simulink model "controlstructureforassignment"  (R2022b)
settings: Solver=ode45  StartTime=0.0  StopTime=300  RelTol=1e-6  EnableMultiTasking=on
values from neighbouring files (symbols this model uses):
  At = 63.6    [LAB.m]
  h10 = 14    [LAB.m]
  h20 = 14    [LAB.m]
  K_q = 10    [LAB.m]
  Ki = Tau/(Kp*lambda)    [LAB.m]
  Kp = 0.1572*Tau    (= 7.09706546275)    [LAB.m]
  Kr = 1    [LAB.m]
  Lc = 1    [LAB.m]
  point = [14, 14]    [LAB.m]
  u10 = u_1_init    [LAB.m]
  u20 = u_2_init    [LAB.m]
settings Model: Creator=magni246  LastModifiedBy=danisode
settings SolverCC: ZeroCrossAlgorithm=Non-adaptive  AlgebraicLoopSolver=TrustRegion
settings DataIOCC: LimitDataPoints=on  SaveFormat=Array  SignalLoggingSaveFormat=ModelDataLogs  ReturnWorkspaceOutputs=off
settings OptimizationCC: ExpressionDepthLimit=2147483647  InitFltsAndDblsToZero=on  LifeSpan=inf
settings DebuggingCC: UnderspecifiedInitializationDetection=Classic  MergeDetectMultiDrivingBlocksExec=none  SolverPrmCheckMsg=warning  FcnCallInpInsideContextMsg=warning  UnconnectedInputMsg=warning  UnconnectedOutputMsg=warning  UnconnectedLineMsg=warning  StateNameClashWarn=warning  SFUnexpectedBacktrackingDiag=warning  SFNoUnconditionalDefaultTransitionDiag=warning  SFExecutionAtInitializationDiag=none  SFMachineParentedDataDiag=warning  ArithmeticOperatorsInVariantConditions=warning
settings HardwareCC: ProdBitPerPointer=32  ProdBitPerSizeT=32  ProdBitPerPtrDiffT=32  ProdLargestAtomicFloat=None  ProdIntDivRoundTo=Undefined  ProdEndianess=Unspecified  ProdWordSize=32  ProdHWDeviceType=32-bit Generic
settings ModelReferenceCC: PropagateSignalLabelsOutOfModel=off
settings CodeAppCC: StateflowObjectComments=on
settings GRTTargetCC: TargetLangStandard=C89/C90 (ANSI)  CombineOutputUpdateFcns=off  GRTInterface=on
settings ConfigComp: CovMetricSettings=dw  CovSaveCumulativeToWorkspaceVar=on  CovSaveSingleToWorkspaceVar=on

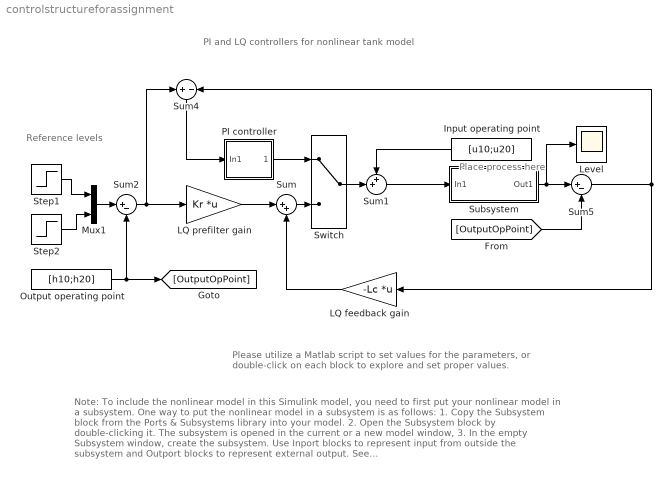
== system controlstructureforassignment ==
  note: Reference
      | levels
  note: Note: To include the nonlinear model in this Simulink model,
      | you need to first put your nonlinear model in a subsystem.
      |
      | One way to put the nonlinear model in a subsystem is as follows:
      |    1.  Copy the Subsystem block from the Ports & Subsystems library into your model.
      |    2. Open the Subsystem block by double-clicking it.
      |       The subsystem is opened in the current or a new model window,
      |    3. In the empty Subsystem window, create the subsystem.
      | Use Inport blocks to represent input from outside the subsystem
      | and Outport blocks to represent external output.
      |
      | See http://www.mathworks.com/access/helpdesk/help/toolbox/simulink/index.html?/access/helpdesk/help/toolbox/simulink/ug/f4-53172.html
  note: Please utilize a Matlab script to set values for the parameters,
      | or double-click on each block to explore and set proper values.
  note: PI and LQ controllers for nonlinear tank model
  note: Place process
      | here
  Input operating point : Constant  Value=[u10;u20]
  LQ feedback gain : Gain  Gain=-Lc  Multiplication=Matrix(K*u)
  LQ prefilter gain : Gain  Gain=Kr  Multiplication=Matrix(K*u)
  Level : Scope
  Mux1 : Mux  Inputs=2
  "Output operating point " : Constant  Value=[h10;h20]
  PI controller : Subsystem
  Step1 : Step  Time=100  Before=h10  After=h10+2  SampleTime=0
  Step2 : Step  Time=100  Before=h20  After=h20  SampleTime=0
  Subsystem : Subsystem
  Sum : Sum  Inputs=|++
  Sum1 : Sum  Inputs=++|
  Sum2 : Sum  Inputs=|+-
  Sum4 : Sum  Inputs=+-
  Sum5 : Sum  Inputs=|+-
  "Switch " : ManualSwitch
  wires:
  LQ prefilter gain/1 -> Sum/1
  LQ feedback gain/1 -> Sum/2
  Sum/1 -> "Switch "/2
  Step2/1 -> Mux1/2
  Step1/1 -> Mux1/1
  Sum1/1 -> Subsystem/1(In1)
  Sum2/1 -> LQ prefilter gain/1, Sum4/1
  Mux1/1 -> Sum2/1
  "Output operating point "/1 -> Sum2/2, [OutputOpPoint]
  PI controller/1(Out1) -> "Switch "/1
  Sum4/1 -> PI controller/1(In1)
  [OutputOpPoint] -> Sum5/2
  Subsystem/1(Out1) -> Sum5/1, Level/1
  Sum5/1 -> LQ feedback gain/1, Sum4/2
  "Switch "/1 -> Sum1/2
  Input operating point/1 -> Sum1/1

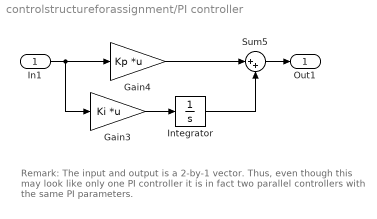
== system controlstructureforassignment/PI controller ==
  note: Remark:  The input and output is a 2-by-1 vector.  Thus, even though
      | this may look like only one PI controller it is in fact two parallel
      | controllers with the same PI parameters.
  In1 : Inport
  Gain3 : Gain  Gain=Ki  Multiplication=Matrix(K*u)
  Gain4 : Gain  Gain=Kp  Multiplication=Matrix(K*u)
  Integrator : Integrator  LimitOutput=on  UpperSaturationLimit=10  LowerSaturationLimit=-10
  Sum5 : Sum  Inputs=|++
  Out1 : Outport
  wires:
  In1/1 -> Gain4/1, Gain3/1
  Gain4/1 -> Sum5/1
  Sum5/1 -> Out1/1
  Integrator/1 -> Sum5/2
  Gain3/1 -> Integrator/1

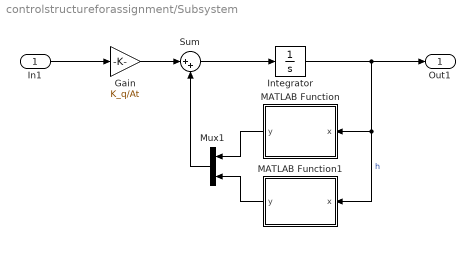
== system controlstructureforassignment/Subsystem ==
  In1 : Inport
  Gain : Gain  Gain=K_q/At
  Integrator : Integrator  InitialCondition=point
  MATLAB Function : MATLAB Function  TreatAsAtomicUnit=on
  MATLAB Function1 : MATLAB Function  TreatAsAtomicUnit=on
  Mux1 : Mux  Inputs=2
  Sum : Sum  Inputs=|++
  Out1 : Outport
  wires:
  Integrator/1 -> Out1/1, MATLAB Function1/1(x), MATLAB Function/1(x)  "h"
  In1/1 -> Gain/1
  Mux1/1 -> Sum/2
  MATLAB Function1/1(y) -> Mux1/2
  MATLAB Function/1(y) -> Mux1/1
  Gain/1 -> Sum/1
  Sum/1 -> Integrator/1

== matlab function controlstructureforassignment/Subsystem/MATLAB Function1 ==
  data: x input; y output
function y = fcn(x)
h_1 = x(1);
h_2 = x(2);
y = (5*h_1)/53 - (5*h_2)/53 - (119*218^(1/2)*h_2^(1/2))/10600;

== matlab function controlstructureforassignment/Subsystem/MATLAB Function ==
  data: x input; y output
function y = fcn(x)
h_1 = x(1);
h_2 = x(2);
y = (5*h_2)/53 - (5*h_1)/53 - (119*218^(1/2)*h_1^(1/2))/10600;
